simulink model "Final_IHA_2706_2015a"  (R2016b)
settings: Solver=ode5  StartTime=0.0  StopTime=20  FixedStep=SampleTime  RelTol=1e-3  EnableMultiTasking=on
values from neighbouring files (symbols this model uses):
  K = 2000    [code_final.m]
  PowerOn = 0    [code_final.m]
  q = 41.3    [code_final.m]
  Q_AT_break = [-1 -0.7 -0.5 -0.3 -0.2 -0.1 0 0.2 0.8 1]    [code_final.m]
  Q_AT_look = [1 0.1991 0.1227 0.07575 0.04002 0.01761 0.00075 5.86e-8 5.86e-8 5.86e-8]    [code_final.m]
  Q_BT_break = [-1 -0.6 -0.2 0 0.1 0.2 0.3 0.4 0.5 1]    [code_final.m]
  Q_BT_look = [5.86e-8 5.86e-8 5.86e-8 0.000913 0.02175 0.040 0.081 0.10 0.20 1]    [code_final.m]
  Q_PA_break = [-1 -0.6 -0.2 0 0.1 0.2 0.3 0.4 0.5 1]    [code_final.m]
  Q_PA_look = [5.86e-8 5.86e-8 5.86e-8 0.000876 0.0214 0.044 0.071 0.1 0.15 1]    [code_final.m]
  Q_PB_break = [-1 -0.7 -0.5 -0.3 -0.2 -0.1 0 0.2 0.8 1]    [code_final.m]
  Q_PB_look = [1 0.1498 0.1 0.077 0.03591 0.021 0.00082 5.86e-8 5.86e-8 5.86e-8]    [code_final.m]
  SampleTime = .001    (= 0.001)    [code_final.m]
undefined symbols (not defined in the file or in its folder): b, Cylinder, Cylinder1, Cylinder2, Cylinder3, Cylinder4, DiscIntNeverNeededParam, FC, FL1, FL2, FS, Lift, Pillar, Pinion, Piston, Rack, tilt, Valve, VS, X, X1, X2, Y, Z
undefined symbols (not defined in the file): Cyl, HoseA, HoseB, Valve2, Valve3, Valve4
libraries: sm_lib x67, simulink x32, nesl_utility x20, simulink_extras x3, xpcrtudplib x2, xpcobsoletelib x2
(part 4 of 4)

== system Final_IHA_2706_2015a/hydraulics/Cylinder3/Valve System3/Relative openings ==
  Spool_position : Inport
  1-D Lookup Table : Lookup_n-D  NumberOfTableDimensions=1  BreakpointsForDimension1=Q_PA_break  Table=Q_PA_look  InternalRulePriority=Speed  RndMeth=Simplest  InputSameDT=on
  1-D Lookup Table1 : Lookup_n-D  NumberOfTableDimensions=1  BreakpointsForDimension1=Q_PB_break  Table=Q_PB_look  InternalRulePriority=Speed  RndMeth=Simplest  InputSameDT=on
  1-D Lookup Table2 : Lookup_n-D  NumberOfTableDimensions=1  BreakpointsForDimension1=Q_BT_break  Table=Q_BT_look  InternalRulePriority=Speed  RndMeth=Simplest  InputSameDT=on
  1-D Lookup Table3 : Lookup_n-D  NumberOfTableDimensions=1  BreakpointsForDimension1=Q_AT_break  Table=Q_AT_look  InternalRulePriority=Speed  RndMeth=Simplest  InputSameDT=on
  av_PA : Outport
  av_PB : Outport  Port=2
  av_BT : Outport  Port=3
  av_AT : Outport  Port=4
  wires:
  1-D Lookup Table3/1 -> av_AT/1
  1-D Lookup Table/1 -> av_PA/1
  1-D Lookup Table2/1 -> av_BT/1
  1-D Lookup Table1/1 -> av_PB/1
  Spool_position/1 -> 1-D Lookup Table3/1, 1-D Lookup Table1/1, 1-D Lookup Table2/1, 1-D Lookup Table/1

== system Final_IHA_2706_2015a/hydraulics/Cylinder3/Valve System3/Valve Dynamics ==
  Control [-1....1] : Inport
  Saturation1 : Saturate  UpperLimit=1  LowerLimit=-1
  Transfer Fcn1 : TransferFcn  Numerator=[q^2]  Denominator=[1 2*t*q q^2]
  Transport Delay1 : TransportDelay  DelayTime=Valve.delay
  Spool Position [-1....1] : Outport
  wires:
  Transport Delay1/1 -> Transfer Fcn1/1
  Transfer Fcn1/1 -> Saturation1/1
  Control [-1....1]/1 -> Transport Delay1/1
  Saturation1/1 -> Spool Position [-1....1]/1

== system Final_IHA_2706_2015a/hydraulics/Cylinder4/Cylinder4/Chamber A ==
  Q_in : Inport
  " V" : Inport  Port=2
  " dV/dt" : Inport  Port=3
  " B" : Inport  Port=4
  Integrator : Integrator  InitialCondition=pinitial  AbsoluteTolerance=10
  Product : Product  Inputs=*/*  SaturateOnIntegerOverflow=on  InputSameDT=on  OutDataTypeStr=Inherit: Same as first input
  Saturation : Saturate  UpperLimit=inf  LowerLimit=0
  Sum : Sum  Inputs=+-  SaturateOnIntegerOverflow=on  InputSameDT=on  OutDataTypeStr=Inherit: Same as first input
  p : Outport
  wires:
  Product/1 -> Integrator/1
  Integrator/1 -> Saturation/1
  Saturation/1 -> p/1
  " V"/1 -> Product/2
  " B"/1 -> Product/3
  Q_in/1 -> Sum/1
  " dV/dt"/1 -> Sum/2
  Sum/1 -> Product/1

== system Final_IHA_2706_2015a/hydraulics/Cylinder4/Cylinder4/Chamber B ==
  Q_in : Inport
  " V" : Inport  Port=2
  " dV/dt" : Inport  Port=3
  " B" : Inport  Port=4
  Integrator : Integrator  InitialCondition=pinitial  AbsoluteTolerance=10
  Product : Product  Inputs=*/*  SaturateOnIntegerOverflow=on  InputSameDT=on  OutDataTypeStr=Inherit: Same as first input
  Saturation : Saturate  UpperLimit=inf  LowerLimit=0
  Sum : Sum  Inputs=+-  SaturateOnIntegerOverflow=on  InputSameDT=on  OutDataTypeStr=Inherit: Same as first input
  p : Outport
  wires:
  Product/1 -> Integrator/1
  Integrator/1 -> Saturation/1
  Saturation/1 -> p/1
  " V"/1 -> Product/2
  " B"/1 -> Product/3
  Q_in/1 -> Sum/1
  " dV/dt"/1 -> Sum/2
  Sum/1 -> Product/1

== system Final_IHA_2706_2015a/hydraulics/Cylinder4/Valve System4/Flow paths ==
  av_PA : Inport
  av_BT : Inport  Port=2
  av_PB : Inport  Port=3
  av_AT : Inport  Port=4
  p_A : Inport  Port=5
  p_B : Inport  Port=6
  p_S : Inport  Port=7
  "p_T " : Inport  Port=8
  Add{,1..3} (4 alike) : Sum
  Orifice AT : Subsystem  mask(Hydraulic){QN=Valve4.AT.QN, dpN=Valve4.PA.dpN, ptr=Valve.ptr}
      mask prompts: QN "Nominal Flow [m^3/s] :"; dpN "Nominal Pressure Difference [Pa] :"; ptr "Transition Pressure [Pa] :"
      mask help:
      | Implements numerically robust turbulent flow
      | equation. Polynomial flow equation is used
      | when abs(dp) < Transition Pressure.
      mask init:
      | K = QN/(sqrt(dpN));
      mask Help: eval('hydlibdoc(''orificedoc'')')
  Orifice BT : Subsystem  mask(Hydraulic){QN=Valve4.BT.QN, dpN=Valve4.PA.dpN, ptr=Valve.ptr}
      mask prompts: QN "Nominal Flow [m^3/s] :"; dpN "Nominal Pressure Difference [Pa] :"; ptr "Transition Pressure [Pa] :"
      mask help:
      | Implements numerically robust turbulent flow
      | equation. Polynomial flow equation is used
      | when abs(dp) < Transition Pressure.
      mask init:
      | K = QN/(sqrt(dpN));
      mask Help: eval('hydlibdoc(''orificedoc'')')
  Orifice PA : Subsystem  mask(Hydraulic){QN=Valve4.PA.QN, dpN=Valve4.PA.dpN, ptr=Valve.ptr}
      mask prompts: QN "Nominal Flow [m^3/s] :"; dpN "Nominal Pressure Difference [Pa] :"; ptr "Transition Pressure [Pa] :"
      mask help:
      | Implements numerically robust turbulent flow
      | equation. Polynomial flow equation is used
      | when abs(dp) < Transition Pressure.
      mask init:
      | K = QN/(sqrt(dpN));
      mask Help: eval('hydlibdoc(''orificedoc'')')
  Orifice PB : Subsystem  mask(Hydraulic){QN=Valve4.PB.QN, dpN=Valve4.PA.dpN, ptr=Valve.ptr}
      mask prompts: QN "Nominal Flow [m^3/s] :"; dpN "Nominal Pressure Difference [Pa] :"; ptr "Transition Pressure [Pa] :"
      mask help:
      | Implements numerically robust turbulent flow
      | equation. Polynomial flow equation is used
      | when abs(dp) < Transition Pressure.
      mask init:
      | K = QN/(sqrt(dpN));
      mask Help: eval('hydlibdoc(''orificedoc'')')
  Q_A : Outport
  Q_B : Outport  Port=2
  Q_P : Outport  Port=3
  Q_T : Outport  Port=4
  wires:
  Orifice PB/2(Q_P) -> Add3/2
  Orifice PA/1(Q_P) -> Add3/1
  Add3/1 -> Q_P/1
  Add2/1 -> Q_B/1
  Orifice PB/1(Q_B) -> Add2/2
  Orifice BT/2(Q_B) -> Add2/1
  Add1/1 -> Q_T/1
  Orifice BT/1(Q_T) -> Add1/2
  Orifice AT/2(Q_T) -> Add1/1
  Add/1 -> Q_A/1
  Orifice AT/1(Q_A) -> Add/2
  Orifice PA/2(Q_A) -> Add/1
  av_PB/1 -> Orifice PB/3(u)
  av_AT/1 -> Orifice AT/3(u)
  av_BT/1 -> Orifice BT/3(u)
  av_PA/1 -> Orifice PA/3(u)
  p_B/1 -> Orifice BT/2(p_B), Orifice PB/1(p_B)
  "p_T "/1 -> Orifice AT/2(p_T), Orifice BT/1(p_T)
  p_S/1 -> Orifice PA/1(p_P), Orifice PB/2(p_P)
  p_A/1 -> Orifice PA/2(p_A), Orifice AT/1(p_A)

== system Final_IHA_2706_2015a/hydraulics/Cylinder4/Valve System4/Relative openings ==
  Spool_position : Inport
  1-D Lookup Table : Lookup_n-D  NumberOfTableDimensions=1  BreakpointsForDimension1=Q_PA_break  Table=Q_PA_look  InternalRulePriority=Speed  RndMeth=Simplest  InputSameDT=on
  1-D Lookup Table1 : Lookup_n-D  NumberOfTableDimensions=1  BreakpointsForDimension1=Q_PB_break  Table=Q_PB_look  InternalRulePriority=Speed  RndMeth=Simplest  InputSameDT=on
  1-D Lookup Table2 : Lookup_n-D  NumberOfTableDimensions=1  BreakpointsForDimension1=Q_BT_break  Table=Q_BT_look  InternalRulePriority=Speed  RndMeth=Simplest  InputSameDT=on
  1-D Lookup Table3 : Lookup_n-D  NumberOfTableDimensions=1  BreakpointsForDimension1=Q_AT_break  Table=Q_AT_look  InternalRulePriority=Speed  RndMeth=Simplest  InputSameDT=on
  av_PA : Outport
  av_PB : Outport  Port=2
  av_BT : Outport  Port=3
  av_AT : Outport  Port=4
  wires:
  Spool_position/1 -> 1-D Lookup Table/1, 1-D Lookup Table2/1, 1-D Lookup Table1/1, 1-D Lookup Table3/1
  1-D Lookup Table1/1 -> av_PB/1
  1-D Lookup Table2/1 -> av_BT/1
  1-D Lookup Table/1 -> av_PA/1
  1-D Lookup Table3/1 -> av_AT/1

== system Final_IHA_2706_2015a/hydraulics/Cylinder4/Valve System4/Valve Dynamics ==
  Control [-1....1] : Inport
  Saturation1 : Saturate  UpperLimit=1  LowerLimit=-1
  Transfer Fcn1 : TransferFcn  Numerator=[q^2]  Denominator=[1 2*t*q q^2]
  Transport Delay1 : TransportDelay  DelayTime=Valve.delay
  Spool Position [-1....1] : Outport
  wires:
  Saturation1/1 -> Spool Position [-1....1]/1
  Control [-1....1]/1 -> Transport Delay1/1
  Transfer Fcn1/1 -> Saturation1/1
  Transport Delay1/1 -> Transfer Fcn1/1

== system Final_IHA_2706_2015a/hydraulics/Cylinder1/Valve System1/Flow paths/Orifice AT ==
  p_A : Inport
  p_T : Inport  Port=2
  u : Inport  Port=3
  Abs : Abs  ZeroCross=off  SaturateOnIntegerOverflow=on
  Add : Sum  Inputs=+-
  Fcn : Fcn  Expr=u[2]*u[1]/2.0/sqrt(ptr)*(3-u[1]/ptr)
  Fcn-Saturation : Fcn  Expr=(u(1)>=-1e-10)*u(1)
  Gain : Gain  Gain=K  SaturateOnIntegerOverflow=on  OutDataTypeStr=Inherit: Same as input  ParamDataTypeStr=Inherit: Same as input
  Gain1 : Gain  Gain=-1  SaturateOnIntegerOverflow=on  OutDataTypeStr=Inherit: Same as input  ParamDataTypeStr=Inherit: Same as input
  Math Function1 : Math  Operator=sqrt  SaturateOnIntegerOverflow=on
  Mux : Mux  Inputs=2
  Product : Product  SaturateOnIntegerOverflow=on  InputSameDT=on  OutDataTypeStr=Inherit: Same as first input
  Product1 : Product  SaturateOnIntegerOverflow=on  InputSameDT=on  OutDataTypeStr=Inherit: Same as first input
  Sign : Signum  ZeroCross=off
  "Switch, treshold = ptr" : Switch  Threshold=ptr  ZeroCross=off  SaturateOnIntegerOverflow=on
  Q_A : Outport  InitialOutput=0
  Q_T : Outport  Port=2  InitialOutput=0
  wires:
  u/1 -> Fcn-Saturation/1
  Fcn/1 -> "Switch, treshold = ptr"/3
  Mux/1 -> Fcn/1
  Product/1 -> "Switch, treshold = ptr"/1
  Math Function1/1 -> Product/1
  Abs/1 -> "Switch, treshold = ptr"/2, Mux/1, Math Function1/1
  Fcn-Saturation/1 -> Gain/1
  Gain/1 -> Product/2, Mux/2
  "Switch, treshold = ptr"/1 -> Product1/2
  Sign/1 -> Product1/1
  p_A/1 -> Add/1
  p_T/1 -> Add/2
  Add/1 -> Abs/1, Sign/1
  Product1/1 -> Q_T/1, Gain1/1
  Gain1/1 -> Q_A/1

== system Final_IHA_2706_2015a/hydraulics/Cylinder1/Valve System1/Flow paths/Orifice BT ==
  p_T : Inport
  p_B : Inport  Port=2
  u : Inport  Port=3
  Abs : Abs  ZeroCross=off  SaturateOnIntegerOverflow=on
  Add : Sum  Inputs=+-
  Fcn : Fcn  Expr=u[2]*u[1]/2.0/sqrt(ptr)*(3-u[1]/ptr)
  Fcn-Saturation : Fcn  Expr=(u(1)>=-1e-10)*u(1)
  Gain : Gain  Gain=K  SaturateOnIntegerOverflow=on  OutDataTypeStr=Inherit: Same as input  ParamDataTypeStr=Inherit: Same as input
  Gain1 : Gain  Gain=-1  SaturateOnIntegerOverflow=on  OutDataTypeStr=Inherit: Same as input  ParamDataTypeStr=Inherit: Same as input
  Math Function1 : Math  Operator=sqrt  SaturateOnIntegerOverflow=on
  Mux : Mux  Inputs=2
  Product : Product  SaturateOnIntegerOverflow=on  InputSameDT=on  OutDataTypeStr=Inherit: Same as first input
  Product1 : Product  SaturateOnIntegerOverflow=on  InputSameDT=on  OutDataTypeStr=Inherit: Same as first input
  Sign : Signum  ZeroCross=off
  "Switch, treshold = ptr" : Switch  Threshold=ptr  ZeroCross=off  SaturateOnIntegerOverflow=on
  Q_T : Outport  InitialOutput=0
  Q_B : Outport  Port=2  InitialOutput=0
  wires:
  Gain1/1 -> Q_T/1
  Product1/1 -> Gain1/1, Q_B/1
  Add/1 -> Sign/1, Abs/1
  p_B/1 -> Add/2
  p_T/1 -> Add/1
  Sign/1 -> Product1/1
  "Switch, treshold = ptr"/1 -> Product1/2
  Gain/1 -> Mux/2, Product/2
  Fcn-Saturation/1 -> Gain/1
  Abs/1 -> Math Function1/1, Mux/1, "Switch, treshold = ptr"/2
  Math Function1/1 -> Product/1
  Product/1 -> "Switch, treshold = ptr"/1
  Mux/1 -> Fcn/1
  Fcn/1 -> "Switch, treshold = ptr"/3
  u/1 -> Fcn-Saturation/1

== system Final_IHA_2706_2015a/hydraulics/Cylinder1/Valve System1/Flow paths/Orifice PA ==
  p_P : Inport
  p_A : Inport  Port=2
  u : Inport  Port=3
  Abs : Abs  ZeroCross=off  SaturateOnIntegerOverflow=on
  Add : Sum  Inputs=+-
  Fcn : Fcn  Expr=u[2]*u[1]/2.0/sqrt(ptr)*(3-u[1]/ptr)
  Fcn-Saturation : Fcn  Expr=(u(1)>=-1e-10)*u(1)
  Gain : Gain  Gain=K  SaturateOnIntegerOverflow=on  OutDataTypeStr=Inherit: Same as input  ParamDataTypeStr=Inherit: Same as input
  Gain1 : Gain  Gain=-1  SaturateOnIntegerOverflow=on  OutDataTypeStr=Inherit: Same as input  ParamDataTypeStr=Inherit: Same as input
  Math Function1 : Math  Operator=sqrt  SaturateOnIntegerOverflow=on
  Mux : Mux  Inputs=2
  Product : Product  SaturateOnIntegerOverflow=on  InputSameDT=on  OutDataTypeStr=Inherit: Same as first input
  Product1 : Product  SaturateOnIntegerOverflow=on  InputSameDT=on  OutDataTypeStr=Inherit: Same as first input
  Sign : Signum  ZeroCross=off
  "Switch, treshold = ptr" : Switch  Threshold=ptr  ZeroCross=off  SaturateOnIntegerOverflow=on
  Q_P : Outport  InitialOutput=0
  Q_A : Outport  Port=2  InitialOutput=0
  wires:
  u/1 -> Fcn-Saturation/1
  Fcn/1 -> "Switch, treshold = ptr"/3
  Mux/1 -> Fcn/1
  Product/1 -> "Switch, treshold = ptr"/1
  Math Function1/1 -> Product/1
  Abs/1 -> "Switch, treshold = ptr"/2, Mux/1, Math Function1/1
  Fcn-Saturation/1 -> Gain/1
  Gain/1 -> Product/2, Mux/2
  "Switch, treshold = ptr"/1 -> Product1/2
  Sign/1 -> Product1/1
  p_P/1 -> Add/1
  p_A/1 -> Add/2
  Add/1 -> Abs/1, Sign/1
  Product1/1 -> Q_A/1, Gain1/1
  Gain1/1 -> Q_P/1

== system Final_IHA_2706_2015a/hydraulics/Cylinder1/Valve System1/Flow paths/Orifice PB ==
  p_B : Inport
  p_P : Inport  Port=2
  u : Inport  Port=3
  Abs : Abs  ZeroCross=off  SaturateOnIntegerOverflow=on
  Add : Sum  Inputs=+-
  Fcn : Fcn  Expr=u[2]*u[1]/2.0/sqrt(ptr)*(3-u[1]/ptr)
  Fcn-Saturation : Fcn  Expr=(u(1)>=-1e-10)*u(1)
  Gain : Gain  Gain=K  SaturateOnIntegerOverflow=on  OutDataTypeStr=Inherit: Same as input  ParamDataTypeStr=Inherit: Same as input
  Gain1 : Gain  Gain=-1  SaturateOnIntegerOverflow=on  OutDataTypeStr=Inherit: Same as input  ParamDataTypeStr=Inherit: Same as input
  Math Function1 : Math  Operator=sqrt  SaturateOnIntegerOverflow=on
  Mux : Mux  Inputs=2
  Product : Product  SaturateOnIntegerOverflow=on  InputSameDT=on  OutDataTypeStr=Inherit: Same as first input
  Product1 : Product  SaturateOnIntegerOverflow=on  InputSameDT=on  OutDataTypeStr=Inherit: Same as first input
  Sign : Signum  ZeroCross=off
  "Switch, treshold = ptr" : Switch  Threshold=ptr  ZeroCross=off  SaturateOnIntegerOverflow=on
  Q_B : Outport  InitialOutput=0
  Q_P : Outport  Port=2  InitialOutput=0
  wires:
  Gain1/1 -> Q_B/1
  Product1/1 -> Gain1/1, Q_P/1
  Add/1 -> Sign/1, Abs/1
  p_P/1 -> Add/2
  p_B/1 -> Add/1
  Sign/1 -> Product1/1
  "Switch, treshold = ptr"/1 -> Product1/2
  Gain/1 -> Mux/2, Product/2
  Fcn-Saturation/1 -> Gain/1
  Abs/1 -> Math Function1/1, Mux/1, "Switch, treshold = ptr"/2
  Math Function1/1 -> Product/1
  Product/1 -> "Switch, treshold = ptr"/1
  Mux/1 -> Fcn/1
  Fcn/1 -> "Switch, treshold = ptr"/3
  u/1 -> Fcn-Saturation/1

== system Final_IHA_2706_2015a/hydraulics/Cylinder2/Valve System2/Flow paths/Orifice AT ==
  p_A : Inport
  p_T : Inport  Port=2
  u : Inport  Port=3
  Abs : Abs  ZeroCross=off  SaturateOnIntegerOverflow=on
  Add : Sum  Inputs=+-
  Fcn : Fcn  Expr=u[2]*u[1]/2.0/sqrt(ptr)*(3-u[1]/ptr)
  Fcn-Saturation : Fcn  Expr=(u(1)>=-1e-10)*u(1)
  Gain : Gain  Gain=K  SaturateOnIntegerOverflow=on  OutDataTypeStr=Inherit: Same as input  ParamDataTypeStr=Inherit: Same as input
  Gain1 : Gain  Gain=-1  SaturateOnIntegerOverflow=on  OutDataTypeStr=Inherit: Same as input  ParamDataTypeStr=Inherit: Same as input
  Math Function1 : Math  Operator=sqrt  SaturateOnIntegerOverflow=on
  Mux : Mux  Inputs=2
  Product : Product  SaturateOnIntegerOverflow=on  InputSameDT=on  OutDataTypeStr=Inherit: Same as first input
  Product1 : Product  SaturateOnIntegerOverflow=on  InputSameDT=on  OutDataTypeStr=Inherit: Same as first input
  Sign : Signum  ZeroCross=off
  "Switch, treshold = ptr" : Switch  Threshold=ptr  ZeroCross=off  SaturateOnIntegerOverflow=on
  Q_A : Outport  InitialOutput=0
  Q_T : Outport  Port=2  InitialOutput=0
  wires:
  Gain1/1 -> Q_A/1
  Product1/1 -> Gain1/1, Q_T/1
  Add/1 -> Sign/1, Abs/1
  p_T/1 -> Add/2
  p_A/1 -> Add/1
  Sign/1 -> Product1/1
  "Switch, treshold = ptr"/1 -> Product1/2
  Gain/1 -> Mux/2, Product/2
  Fcn-Saturation/1 -> Gain/1
  Abs/1 -> Math Function1/1, Mux/1, "Switch, treshold = ptr"/2
  Math Function1/1 -> Product/1
  Product/1 -> "Switch, treshold = ptr"/1
  Mux/1 -> Fcn/1
  Fcn/1 -> "Switch, treshold = ptr"/3
  u/1 -> Fcn-Saturation/1

== system Final_IHA_2706_2015a/hydraulics/Cylinder2/Valve System2/Flow paths/Orifice BT ==
  p_T : Inport
  p_B : Inport  Port=2
  u : Inport  Port=3
  Abs : Abs  ZeroCross=off  SaturateOnIntegerOverflow=on
  Add : Sum  Inputs=+-
  Fcn : Fcn  Expr=u[2]*u[1]/2.0/sqrt(ptr)*(3-u[1]/ptr)
  Fcn-Saturation : Fcn  Expr=(u(1)>=-1e-10)*u(1)
  Gain : Gain  Gain=K  SaturateOnIntegerOverflow=on  OutDataTypeStr=Inherit: Same as input  ParamDataTypeStr=Inherit: Same as input
  Gain1 : Gain  Gain=-1  SaturateOnIntegerOverflow=on  OutDataTypeStr=Inherit: Same as input  ParamDataTypeStr=Inherit: Same as input
  Math Function1 : Math  Operator=sqrt  SaturateOnIntegerOverflow=on
  Mux : Mux  Inputs=2
  Product : Product  SaturateOnIntegerOverflow=on  InputSameDT=on  OutDataTypeStr=Inherit: Same as first input
  Product1 : Product  SaturateOnIntegerOverflow=on  InputSameDT=on  OutDataTypeStr=Inherit: Same as first input
  Sign : Signum  ZeroCross=off
  "Switch, treshold = ptr" : Switch  Threshold=ptr  ZeroCross=off  SaturateOnIntegerOverflow=on
  Q_T : Outport  InitialOutput=0
  Q_B : Outport  Port=2  InitialOutput=0
  wires:
  u/1 -> Fcn-Saturation/1
  Fcn/1 -> "Switch, treshold = ptr"/3
  Mux/1 -> Fcn/1
  Product/1 -> "Switch, treshold = ptr"/1
  Math Function1/1 -> Product/1
  Abs/1 -> "Switch, treshold = ptr"/2, Mux/1, Math Function1/1
  Fcn-Saturation/1 -> Gain/1
  Gain/1 -> Product/2, Mux/2
  "Switch, treshold = ptr"/1 -> Product1/2
  Sign/1 -> Product1/1
  p_T/1 -> Add/1
  p_B/1 -> Add/2
  Add/1 -> Abs/1, Sign/1
  Product1/1 -> Q_B/1, Gain1/1
  Gain1/1 -> Q_T/1

== system Final_IHA_2706_2015a/hydraulics/Cylinder2/Valve System2/Flow paths/Orifice PA ==
  p_P : Inport
  p_A : Inport  Port=2
  u : Inport  Port=3
  Abs : Abs  ZeroCross=off  SaturateOnIntegerOverflow=on
  Add : Sum  Inputs=+-
  Fcn : Fcn  Expr=u[2]*u[1]/2.0/sqrt(ptr)*(3-u[1]/ptr)
  Fcn-Saturation : Fcn  Expr=(u(1)>=-1e-10)*u(1)
  Gain : Gain  Gain=K  SaturateOnIntegerOverflow=on  OutDataTypeStr=Inherit: Same as input  ParamDataTypeStr=Inherit: Same as input
  Gain1 : Gain  Gain=-1  SaturateOnIntegerOverflow=on  OutDataTypeStr=Inherit: Same as input  ParamDataTypeStr=Inherit: Same as input
  Math Function1 : Math  Operator=sqrt  SaturateOnIntegerOverflow=on
  Mux : Mux  Inputs=2
  Product : Product  SaturateOnIntegerOverflow=on  InputSameDT=on  OutDataTypeStr=Inherit: Same as first input
  Product1 : Product  SaturateOnIntegerOverflow=on  InputSameDT=on  OutDataTypeStr=Inherit: Same as first input
  Sign : Signum  ZeroCross=off
  "Switch, treshold = ptr" : Switch  Threshold=ptr  ZeroCross=off  SaturateOnIntegerOverflow=on
  Q_P : Outport  InitialOutput=0
  Q_A : Outport  Port=2  InitialOutput=0
  wires:
  Gain1/1 -> Q_P/1
  Product1/1 -> Gain1/1, Q_A/1
  Add/1 -> Sign/1, Abs/1
  p_A/1 -> Add/2
  p_P/1 -> Add/1
  Sign/1 -> Product1/1
  "Switch, treshold = ptr"/1 -> Product1/2
  Gain/1 -> Mux/2, Product/2
  Fcn-Saturation/1 -> Gain/1
  Abs/1 -> Math Function1/1, Mux/1, "Switch, treshold = ptr"/2
  Math Function1/1 -> Product/1
  Product/1 -> "Switch, treshold = ptr"/1
  Mux/1 -> Fcn/1
  Fcn/1 -> "Switch, treshold = ptr"/3
  u/1 -> Fcn-Saturation/1

== system Final_IHA_2706_2015a/hydraulics/Cylinder2/Valve System2/Flow paths/Orifice PB ==
  p_B : Inport
  p_P : Inport  Port=2
  u : Inport  Port=3
  Abs : Abs  ZeroCross=off  SaturateOnIntegerOverflow=on
  Add : Sum  Inputs=+-
  Fcn : Fcn  Expr=u[2]*u[1]/2.0/sqrt(ptr)*(3-u[1]/ptr)
  Fcn-Saturation : Fcn  Expr=(u(1)>=-1e-10)*u(1)
  Gain : Gain  Gain=K  SaturateOnIntegerOverflow=on  OutDataTypeStr=Inherit: Same as input  ParamDataTypeStr=Inherit: Same as input
  Gain1 : Gain  Gain=-1  SaturateOnIntegerOverflow=on  OutDataTypeStr=Inherit: Same as input  ParamDataTypeStr=Inherit: Same as input
  Math Function1 : Math  Operator=sqrt  SaturateOnIntegerOverflow=on
  Mux : Mux  Inputs=2
  Product : Product  SaturateOnIntegerOverflow=on  InputSameDT=on  OutDataTypeStr=Inherit: Same as first input
  Product1 : Product  SaturateOnIntegerOverflow=on  InputSameDT=on  OutDataTypeStr=Inherit: Same as first input
  Sign : Signum  ZeroCross=off
  "Switch, treshold = ptr" : Switch  Threshold=ptr  ZeroCross=off  SaturateOnIntegerOverflow=on
  Q_B : Outport  InitialOutput=0
  Q_P : Outport  Port=2  InitialOutput=0
  wires:
  u/1 -> Fcn-Saturation/1
  Fcn/1 -> "Switch, treshold = ptr"/3
  Mux/1 -> Fcn/1
  Product/1 -> "Switch, treshold = ptr"/1
  Math Function1/1 -> Product/1
  Abs/1 -> "Switch, treshold = ptr"/2, Mux/1, Math Function1/1
  Fcn-Saturation/1 -> Gain/1
  Gain/1 -> Product/2, Mux/2
  "Switch, treshold = ptr"/1 -> Product1/2
  Sign/1 -> Product1/1
  p_B/1 -> Add/1
  p_P/1 -> Add/2
  Add/1 -> Abs/1, Sign/1
  Product1/1 -> Q_P/1, Gain1/1
  Gain1/1 -> Q_B/1

== system Final_IHA_2706_2015a/hydraulics/Cylinder3/Valve System3/Flow paths/Orifice AT ==
  p_A : Inport
  p_T : Inport  Port=2
  u : Inport  Port=3
  Abs : Abs  ZeroCross=off  SaturateOnIntegerOverflow=on
  Add : Sum  Inputs=+-
  Fcn : Fcn  Expr=u[2]*u[1]/2.0/sqrt(ptr)*(3-u[1]/ptr)
  Fcn-Saturation : Fcn  Expr=(u(1)>=-1e-10)*u(1)
  Gain : Gain  Gain=K  SaturateOnIntegerOverflow=on  OutDataTypeStr=Inherit: Same as input  ParamDataTypeStr=Inherit: Same as input
  Gain1 : Gain  Gain=-1  SaturateOnIntegerOverflow=on  OutDataTypeStr=Inherit: Same as input  ParamDataTypeStr=Inherit: Same as input
  Math Function1 : Math  Operator=sqrt  SaturateOnIntegerOverflow=on
  Mux : Mux  Inputs=2
  Product : Product  SaturateOnIntegerOverflow=on  InputSameDT=on  OutDataTypeStr=Inherit: Same as first input
  Product1 : Product  SaturateOnIntegerOverflow=on  InputSameDT=on  OutDataTypeStr=Inherit: Same as first input
  Sign : Signum  ZeroCross=off
  "Switch, treshold = ptr" : Switch  Threshold=ptr  ZeroCross=off  SaturateOnIntegerOverflow=on
  Q_A : Outport  InitialOutput=0
  Q_T : Outport  Port=2  InitialOutput=0
  wires:
  u/1 -> Fcn-Saturation/1
  Fcn/1 -> "Switch, treshold = ptr"/3
  Mux/1 -> Fcn/1
  Product/1 -> "Switch, treshold = ptr"/1
  Math Function1/1 -> Product/1
  Abs/1 -> "Switch, treshold = ptr"/2, Mux/1, Math Function1/1
  Fcn-Saturation/1 -> Gain/1
  Gain/1 -> Product/2, Mux/2
  "Switch, treshold = ptr"/1 -> Product1/2
  Sign/1 -> Product1/1
  p_A/1 -> Add/1
  p_T/1 -> Add/2
  Add/1 -> Abs/1, Sign/1
  Product1/1 -> Q_T/1, Gain1/1
  Gain1/1 -> Q_A/1

== system Final_IHA_2706_2015a/hydraulics/Cylinder3/Valve System3/Flow paths/Orifice BT ==
  p_T : Inport
  p_B : Inport  Port=2
  u : Inport  Port=3
  Abs : Abs  ZeroCross=off  SaturateOnIntegerOverflow=on
  Add : Sum  Inputs=+-
  Fcn : Fcn  Expr=u[2]*u[1]/2.0/sqrt(ptr)*(3-u[1]/ptr)
  Fcn-Saturation : Fcn  Expr=(u(1)>=-1e-10)*u(1)
  Gain : Gain  Gain=K  SaturateOnIntegerOverflow=on  OutDataTypeStr=Inherit: Same as input  ParamDataTypeStr=Inherit: Same as input
  Gain1 : Gain  Gain=-1  SaturateOnIntegerOverflow=on  OutDataTypeStr=Inherit: Same as input  ParamDataTypeStr=Inherit: Same as input
  Math Function1 : Math  Operator=sqrt  SaturateOnIntegerOverflow=on
  Mux : Mux  Inputs=2
  Product : Product  SaturateOnIntegerOverflow=on  InputSameDT=on  OutDataTypeStr=Inherit: Same as first input
  Product1 : Product  SaturateOnIntegerOverflow=on  InputSameDT=on  OutDataTypeStr=Inherit: Same as first input
  Sign : Signum  ZeroCross=off
  "Switch, treshold = ptr" : Switch  Threshold=ptr  ZeroCross=off  SaturateOnIntegerOverflow=on
  Q_T : Outport  InitialOutput=0
  Q_B : Outport  Port=2  InitialOutput=0
  wires:
  Gain1/1 -> Q_T/1
  Product1/1 -> Gain1/1, Q_B/1
  Add/1 -> Sign/1, Abs/1
  p_B/1 -> Add/2
  p_T/1 -> Add/1
  Sign/1 -> Product1/1
  "Switch, treshold = ptr"/1 -> Product1/2
  Gain/1 -> Mux/2, Product/2
  Fcn-Saturation/1 -> Gain/1
  Abs/1 -> Math Function1/1, Mux/1, "Switch, treshold = ptr"/2
  Math Function1/1 -> Product/1
  Product/1 -> "Switch, treshold = ptr"/1
  Mux/1 -> Fcn/1
  Fcn/1 -> "Switch, treshold = ptr"/3
  u/1 -> Fcn-Saturation/1

== system Final_IHA_2706_2015a/hydraulics/Cylinder3/Valve System3/Flow paths/Orifice PA ==
  p_P : Inport
  p_A : Inport  Port=2
  u : Inport  Port=3
  Abs : Abs  ZeroCross=off  SaturateOnIntegerOverflow=on
  Add : Sum  Inputs=+-
  Fcn : Fcn  Expr=u[2]*u[1]/2.0/sqrt(ptr)*(3-u[1]/ptr)
  Fcn-Saturation : Fcn  Expr=(u(1)>=-1e-10)*u(1)
  Gain : Gain  Gain=K  SaturateOnIntegerOverflow=on  OutDataTypeStr=Inherit: Same as input  ParamDataTypeStr=Inherit: Same as input
  Gain1 : Gain  Gain=-1  SaturateOnIntegerOverflow=on  OutDataTypeStr=Inherit: Same as input  ParamDataTypeStr=Inherit: Same as input
  Math Function1 : Math  Operator=sqrt  SaturateOnIntegerOverflow=on
  Mux : Mux  Inputs=2
  Product : Product  SaturateOnIntegerOverflow=on  InputSameDT=on  OutDataTypeStr=Inherit: Same as first input
  Product1 : Product  SaturateOnIntegerOverflow=on  InputSameDT=on  OutDataTypeStr=Inherit: Same as first input
  Sign : Signum  ZeroCross=off
  "Switch, treshold = ptr" : Switch  Threshold=ptr  ZeroCross=off  SaturateOnIntegerOverflow=on
  Q_P : Outport  InitialOutput=0
  Q_A : Outport  Port=2  InitialOutput=0
  wires:
  u/1 -> Fcn-Saturation/1
  Fcn/1 -> "Switch, treshold = ptr"/3
  Mux/1 -> Fcn/1
  Product/1 -> "Switch, treshold = ptr"/1
  Math Function1/1 -> Product/1
  Abs/1 -> "Switch, treshold = ptr"/2, Mux/1, Math Function1/1
  Fcn-Saturation/1 -> Gain/1
  Gain/1 -> Product/2, Mux/2
  "Switch, treshold = ptr"/1 -> Product1/2
  Sign/1 -> Product1/1
  p_P/1 -> Add/1
  p_A/1 -> Add/2
  Add/1 -> Abs/1, Sign/1
  Product1/1 -> Q_A/1, Gain1/1
  Gain1/1 -> Q_P/1

== system Final_IHA_2706_2015a/hydraulics/Cylinder3/Valve System3/Flow paths/Orifice PB ==
  p_B : Inport
  p_P : Inport  Port=2
  u : Inport  Port=3
  Abs : Abs  ZeroCross=off  SaturateOnIntegerOverflow=on
  Add : Sum  Inputs=+-
  Fcn : Fcn  Expr=u[2]*u[1]/2.0/sqrt(ptr)*(3-u[1]/ptr)
  Fcn-Saturation : Fcn  Expr=(u(1)>=-1e-10)*u(1)
  Gain : Gain  Gain=K  SaturateOnIntegerOverflow=on  OutDataTypeStr=Inherit: Same as input  ParamDataTypeStr=Inherit: Same as input
  Gain1 : Gain  Gain=-1  SaturateOnIntegerOverflow=on  OutDataTypeStr=Inherit: Same as input  ParamDataTypeStr=Inherit: Same as input
  Math Function1 : Math  Operator=sqrt  SaturateOnIntegerOverflow=on
  Mux : Mux  Inputs=2
  Product : Product  SaturateOnIntegerOverflow=on  InputSameDT=on  OutDataTypeStr=Inherit: Same as first input
  Product1 : Product  SaturateOnIntegerOverflow=on  InputSameDT=on  OutDataTypeStr=Inherit: Same as first input
  Sign : Signum  ZeroCross=off
  "Switch, treshold = ptr" : Switch  Threshold=ptr  ZeroCross=off  SaturateOnIntegerOverflow=on
  Q_B : Outport  InitialOutput=0
  Q_P : Outport  Port=2  InitialOutput=0
  wires:
  Gain1/1 -> Q_B/1
  Product1/1 -> Gain1/1, Q_P/1
  Add/1 -> Sign/1, Abs/1
  p_P/1 -> Add/2
  p_B/1 -> Add/1
  Sign/1 -> Product1/1
  "Switch, treshold = ptr"/1 -> Product1/2
  Gain/1 -> Mux/2, Product/2
  Fcn-Saturation/1 -> Gain/1
  Abs/1 -> Math Function1/1, Mux/1, "Switch, treshold = ptr"/2
  Math Function1/1 -> Product/1
  Product/1 -> "Switch, treshold = ptr"/1
  Mux/1 -> Fcn/1
  Fcn/1 -> "Switch, treshold = ptr"/3
  u/1 -> Fcn-Saturation/1

== system Final_IHA_2706_2015a/hydraulics/Cylinder4/Valve System4/Flow paths/Orifice AT ==
  p_A : Inport
  p_T : Inport  Port=2
  u : Inport  Port=3
  Abs : Abs  ZeroCross=off  SaturateOnIntegerOverflow=on
  Add : Sum  Inputs=+-
  Fcn : Fcn  Expr=u[2]*u[1]/2.0/sqrt(ptr)*(3-u[1]/ptr)
  Fcn-Saturation : Fcn  Expr=(u(1)>=-1e-10)*u(1)
  Gain : Gain  Gain=K  SaturateOnIntegerOverflow=on  OutDataTypeStr=Inherit: Same as input  ParamDataTypeStr=Inherit: Same as input
  Gain1 : Gain  Gain=-1  SaturateOnIntegerOverflow=on  OutDataTypeStr=Inherit: Same as input  ParamDataTypeStr=Inherit: Same as input
  Math Function1 : Math  Operator=sqrt  SaturateOnIntegerOverflow=on
  Mux : Mux  Inputs=2
  Product : Product  SaturateOnIntegerOverflow=on  InputSameDT=on  OutDataTypeStr=Inherit: Same as first input
  Product1 : Product  SaturateOnIntegerOverflow=on  InputSameDT=on  OutDataTypeStr=Inherit: Same as first input
  Sign : Signum  ZeroCross=off
  "Switch, treshold = ptr" : Switch  Threshold=ptr  ZeroCross=off  SaturateOnIntegerOverflow=on
  Q_A : Outport  InitialOutput=0
  Q_T : Outport  Port=2  InitialOutput=0
  wires:
  Gain1/1 -> Q_A/1
  Product1/1 -> Gain1/1, Q_T/1
  Add/1 -> Sign/1, Abs/1
  p_T/1 -> Add/2
  p_A/1 -> Add/1
  Sign/1 -> Product1/1
  "Switch, treshold = ptr"/1 -> Product1/2
  Gain/1 -> Mux/2, Product/2
  Fcn-Saturation/1 -> Gain/1
  Abs/1 -> Math Function1/1, Mux/1, "Switch, treshold = ptr"/2
  Math Function1/1 -> Product/1
  Product/1 -> "Switch, treshold = ptr"/1
  Mux/1 -> Fcn/1
  Fcn/1 -> "Switch, treshold = ptr"/3
  u/1 -> Fcn-Saturation/1

== system Final_IHA_2706_2015a/hydraulics/Cylinder4/Valve System4/Flow paths/Orifice BT ==
  p_T : Inport
  p_B : Inport  Port=2
  u : Inport  Port=3
  Abs : Abs  ZeroCross=off  SaturateOnIntegerOverflow=on
  Add : Sum  Inputs=+-
  Fcn : Fcn  Expr=u[2]*u[1]/2.0/sqrt(ptr)*(3-u[1]/ptr)
  Fcn-Saturation : Fcn  Expr=(u(1)>=-1e-10)*u(1)
  Gain : Gain  Gain=K  SaturateOnIntegerOverflow=on  OutDataTypeStr=Inherit: Same as input  ParamDataTypeStr=Inherit: Same as input
  Gain1 : Gain  Gain=-1  SaturateOnIntegerOverflow=on  OutDataTypeStr=Inherit: Same as input  ParamDataTypeStr=Inherit: Same as input
  Math Function1 : Math  Operator=sqrt  SaturateOnIntegerOverflow=on
  Mux : Mux  Inputs=2
  Product : Product  SaturateOnIntegerOverflow=on  InputSameDT=on  OutDataTypeStr=Inherit: Same as first input
  Product1 : Product  SaturateOnIntegerOverflow=on  InputSameDT=on  OutDataTypeStr=Inherit: Same as first input
  Sign : Signum  ZeroCross=off
  "Switch, treshold = ptr" : Switch  Threshold=ptr  ZeroCross=off  SaturateOnIntegerOverflow=on
  Q_T : Outport  InitialOutput=0
  Q_B : Outport  Port=2  InitialOutput=0
  wires:
  u/1 -> Fcn-Saturation/1
  Fcn/1 -> "Switch, treshold = ptr"/3
  Mux/1 -> Fcn/1
  Product/1 -> "Switch, treshold = ptr"/1
  Math Function1/1 -> Product/1
  Abs/1 -> "Switch, treshold = ptr"/2, Mux/1, Math Function1/1
  Fcn-Saturation/1 -> Gain/1
  Gain/1 -> Product/2, Mux/2
  "Switch, treshold = ptr"/1 -> Product1/2
  Sign/1 -> Product1/1
  p_T/1 -> Add/1
  p_B/1 -> Add/2
  Add/1 -> Abs/1, Sign/1
  Product1/1 -> Q_B/1, Gain1/1
  Gain1/1 -> Q_T/1

== system Final_IHA_2706_2015a/hydraulics/Cylinder4/Valve System4/Flow paths/Orifice PA ==
  p_P : Inport
  p_A : Inport  Port=2
  u : Inport  Port=3
  Abs : Abs  ZeroCross=off  SaturateOnIntegerOverflow=on
  Add : Sum  Inputs=+-
  Fcn : Fcn  Expr=u[2]*u[1]/2.0/sqrt(ptr)*(3-u[1]/ptr)
  Fcn-Saturation : Fcn  Expr=(u(1)>=-1e-10)*u(1)
  Gain : Gain  Gain=K  SaturateOnIntegerOverflow=on  OutDataTypeStr=Inherit: Same as input  ParamDataTypeStr=Inherit: Same as input
  Gain1 : Gain  Gain=-1  SaturateOnIntegerOverflow=on  OutDataTypeStr=Inherit: Same as input  ParamDataTypeStr=Inherit: Same as input
  Math Function1 : Math  Operator=sqrt  SaturateOnIntegerOverflow=on
  Mux : Mux  Inputs=2
  Product : Product  SaturateOnIntegerOverflow=on  InputSameDT=on  OutDataTypeStr=Inherit: Same as first input
  Product1 : Product  SaturateOnIntegerOverflow=on  InputSameDT=on  OutDataTypeStr=Inherit: Same as first input
  Sign : Signum  ZeroCross=off
  "Switch, treshold = ptr" : Switch  Threshold=ptr  ZeroCross=off  SaturateOnIntegerOverflow=on
  Q_P : Outport  InitialOutput=0
  Q_A : Outport  Port=2  InitialOutput=0
  wires:
  Gain1/1 -> Q_P/1
  Product1/1 -> Gain1/1, Q_A/1
  Add/1 -> Sign/1, Abs/1
  p_A/1 -> Add/2
  p_P/1 -> Add/1
  Sign/1 -> Product1/1
  "Switch, treshold = ptr"/1 -> Product1/2
  Gain/1 -> Mux/2, Product/2
  Fcn-Saturation/1 -> Gain/1
  Abs/1 -> Math Function1/1, Mux/1, "Switch, treshold = ptr"/2
  Math Function1/1 -> Product/1
  Product/1 -> "Switch, treshold = ptr"/1
  Mux/1 -> Fcn/1
  Fcn/1 -> "Switch, treshold = ptr"/3
  u/1 -> Fcn-Saturation/1

== system Final_IHA_2706_2015a/hydraulics/Cylinder4/Valve System4/Flow paths/Orifice PB ==
  p_B : Inport
  p_P : Inport  Port=2
  u : Inport  Port=3
  Abs : Abs  ZeroCross=off  SaturateOnIntegerOverflow=on
  Add : Sum  Inputs=+-
  Fcn : Fcn  Expr=u[2]*u[1]/2.0/sqrt(ptr)*(3-u[1]/ptr)
  Fcn-Saturation : Fcn  Expr=(u(1)>=-1e-10)*u(1)
  Gain : Gain  Gain=K  SaturateOnIntegerOverflow=on  OutDataTypeStr=Inherit: Same as input  ParamDataTypeStr=Inherit: Same as input
  Gain1 : Gain  Gain=-1  SaturateOnIntegerOverflow=on  OutDataTypeStr=Inherit: Same as input  ParamDataTypeStr=Inherit: Same as input
  Math Function1 : Math  Operator=sqrt  SaturateOnIntegerOverflow=on
  Mux : Mux  Inputs=2
  Product : Product  SaturateOnIntegerOverflow=on  InputSameDT=on  OutDataTypeStr=Inherit: Same as first input
  Product1 : Product  SaturateOnIntegerOverflow=on  InputSameDT=on  OutDataTypeStr=Inherit: Same as first input
  Sign : Signum  ZeroCross=off
  "Switch, treshold = ptr" : Switch  Threshold=ptr  ZeroCross=off  SaturateOnIntegerOverflow=on
  Q_B : Outport  InitialOutput=0
  Q_P : Outport  Port=2  InitialOutput=0
  wires:
  u/1 -> Fcn-Saturation/1
  Fcn/1 -> "Switch, treshold = ptr"/3
  Mux/1 -> Fcn/1
  Product/1 -> "Switch, treshold = ptr"/1
  Math Function1/1 -> Product/1
  Abs/1 -> "Switch, treshold = ptr"/2, Mux/1, Math Function1/1
  Fcn-Saturation/1 -> Gain/1
  Gain/1 -> Product/2, Mux/2
  "Switch, treshold = ptr"/1 -> Product1/2
  Sign/1 -> Product1/1
  p_B/1 -> Add/1
  p_P/1 -> Add/2
  Add/1 -> Abs/1, Sign/1
  Product1/1 -> Q_P/1, Gain1/1
  Gain1/1 -> Q_B/1
